simulink model "Exp7"  (R2018a)
settings: Solver=VariableStepAuto  StartTime=0.0  StopTime=10.0  RelTol=1e-3
libraries: simulink x3
settings Model: Creator=SHRUTI  LastModifiedBy=SHRUTI

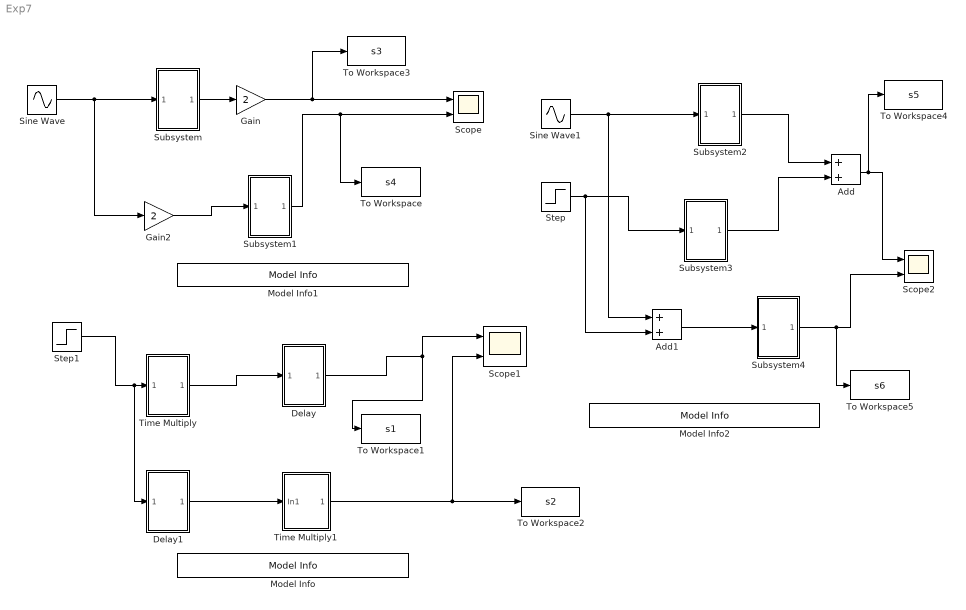
== system Exp7 ==
  Add : Sum
  Add1 : Sum
  Delay : Subsystem
  "Delay1 " : Subsystem
  Gain : Gain  Gain=2
  Gain2 : Gain  Gain=2
  Model Info : simulink/Model-Wide Utilities/Model Info  Frame=on  DisplayStringWithTags=Checking Time Variant/Time Invariant - x(t)cos(wt)  HorizontalTextAlignment=Center  LeftAlignmentValue=0.5
  Model Info1 : simulink/Model-Wide Utilities/Model Info  Frame=on  DisplayStringWithTags=|  HorizontalTextAlignment=Center  LeftAlignmentValue=0.5
      | Checking Linear/NonLinear (Homogineity) -
      |  2x(t) +1
  Model Info2 : simulink/Model-Wide Utilities/Model Info  Frame=on  DisplayStringWithTags="Checking Linear/Non Linear(Additivity) -  2x(t)+1"  HorizontalTextAlignment=Center  LeftAlignmentValue=0.5
  Scope : Scope  NumInputPorts=2
  Scope1 : Scope  NumInputPorts=2
  Scope2 : Scope  NumInputPorts=2
  Sine Wave : Sin  SampleTime=0
  Sine Wave1 : Sin  SampleTime=0
  Step : Step  SampleTime=0
  Step1 : Step  SampleTime=0
  Subsystem : Subsystem
  Subsystem1 : Subsystem
  Subsystem2 : Subsystem
  Subsystem3 : Subsystem
  Subsystem4 : Subsystem
  Time Multiply : Subsystem
  Time Multiply1 : Subsystem
  To Workspace : ToWorkspace  VariableName=s4  SampleTime=-1
  To Workspace1 : ToWorkspace  VariableName=s1  SampleTime=-1
  To Workspace2 : ToWorkspace  VariableName=s2  SampleTime=-1
  To Workspace3 : ToWorkspace  VariableName=s3  SampleTime=-1
  To Workspace4 : ToWorkspace  VariableName=s5  SampleTime=-1
  To Workspace5 : ToWorkspace  VariableName=s6  SampleTime=-1
  wires:
  Step1/1 -> "Delay1 "/1(In1), Time Multiply/1(In1)
  Delay/1(Out1) -> To Workspace1/1, Scope1/1
  Time Multiply/1(Out1) -> Delay/1(In1)
  "Delay1 "/1(Out1) -> Time Multiply1/1(In1)
  Time Multiply1/1(Out1) -> To Workspace2/1, Scope1/2
  Sine Wave/1 -> Gain2/1, Subsystem/1(In1)
  Subsystem/1(Out1) -> Gain/1
  Gain/1 -> To Workspace3/1, Scope/1
  Gain2/1 -> Subsystem1/1(In1)
  Subsystem1/1(Out1) -> To Workspace/1, Scope/2
  Sine Wave1/1 -> Add1/1, Subsystem2/1(In1)
  Step/1 -> Add1/2, Subsystem3/1(In1)
  Subsystem3/1(Out1) -> Add/2
  Subsystem2/1(Out1) -> Add/1
  Add1/1 -> Subsystem4/1(In1)
  Subsystem4/1(Out1) -> To Workspace5/1, Scope2/2
  Add/1 -> To Workspace4/1, Scope2/1

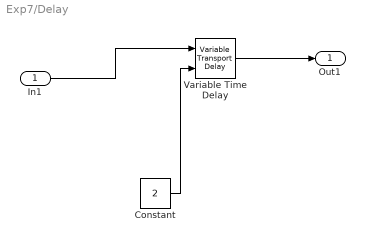
== system Exp7/Delay ==
  In1 : Inport
  Constant : Constant  Value=2
  Variable Time Delay : VariableTransportDelay  MaximumDelay=10
  Out1 : Outport
  wires:
  Constant/1 -> Variable Time Delay/2
  Variable Time Delay/1 -> Out1/1
  In1/1 -> Variable Time Delay/1

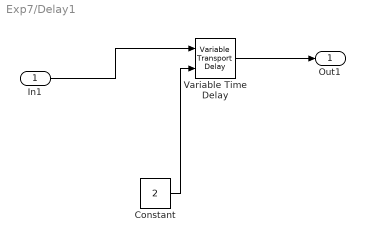
== system Exp7/Delay1  ==
  In1 : Inport
  Constant : Constant  Value=2
  Variable Time Delay : VariableTransportDelay  MaximumDelay=10
  Out1 : Outport
  wires:
  Constant/1 -> Variable Time Delay/2
  Variable Time Delay/1 -> Out1/1
  In1/1 -> Variable Time Delay/1

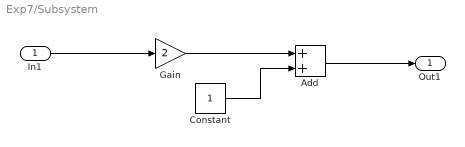
== system Exp7/Subsystem ==
  In1 : Inport
  Add : Sum
  Constant : Constant
  Gain : Gain  Gain=2
  Out1 : Outport
  wires:
  Add/1 -> Out1/1
  Gain/1 -> Add/1
  In1/1 -> Gain/1
  Constant/1 -> Add/2

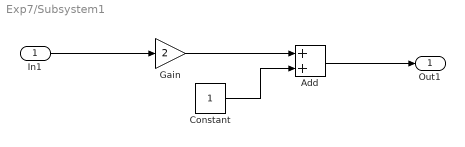
== system Exp7/Subsystem1 ==
  In1 : Inport
  Add : Sum
  Constant : Constant
  Gain : Gain  Gain=2
  Out1 : Outport
  wires:
  Add/1 -> Out1/1
  Gain/1 -> Add/1
  In1/1 -> Gain/1
  Constant/1 -> Add/2

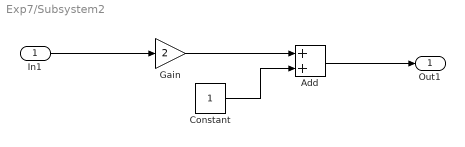
== system Exp7/Subsystem2 ==
  In1 : Inport
  Add : Sum
  Constant : Constant
  Gain : Gain  Gain=2
  Out1 : Outport
  wires:
  Add/1 -> Out1/1
  Gain/1 -> Add/1
  In1/1 -> Gain/1
  Constant/1 -> Add/2

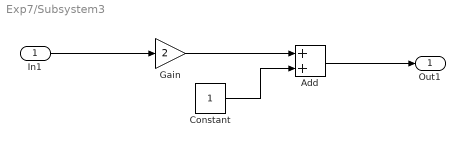
== system Exp7/Subsystem3 ==
  In1 : Inport
  Add : Sum
  Constant : Constant
  Gain : Gain  Gain=2
  Out1 : Outport
  wires:
  Add/1 -> Out1/1
  Gain/1 -> Add/1
  In1/1 -> Gain/1
  Constant/1 -> Add/2

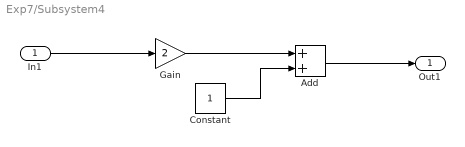
== system Exp7/Subsystem4 ==
  In1 : Inport
  Add : Sum
  Constant : Constant
  Gain : Gain  Gain=2
  Out1 : Outport
  wires:
  Add/1 -> Out1/1
  Gain/1 -> Add/1
  In1/1 -> Gain/1
  Constant/1 -> Add/2

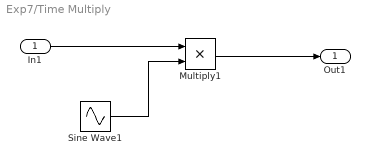
== system Exp7/Time Multiply ==
  In1 : Inport
  Multiply1 : Product
  Sine Wave1 : Sin  SampleTime=0
  Out1 : Outport
  wires:
  Multiply1/1 -> Out1/1
  Sine Wave1/1 -> Multiply1/2
  In1/1 -> Multiply1/1

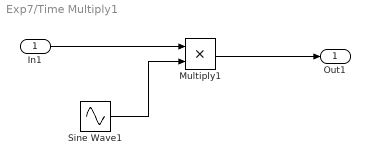
== system Exp7/Time Multiply1 ==
  In1 : Inport
  Multiply1 : Product
  Sine Wave1 : Sin  SampleTime=0
  Out1 : Outport
  wires:
  Multiply1/1 -> Out1/1
  Sine Wave1/1 -> Multiply1/2
  In1/1 -> Multiply1/1
